simulink model "FixedWingModel"  (R2021a)
settings: configuration reference "ctrlConfigSet" (kept outside this file)
values from neighbouring files (symbols this model uses):
  ap = 0.01    [pathFollowingData.sldd]
  env = 0.0065    [pathFollowingData.sldd]
  sensors = 0.0    [pathFollowingData.sldd]
  uavParam = 2.795    [pathFollowingData.sldd]
undefined symbols (not defined in the file or in its folder): DiscIntNeverNeededParam, Earth, WGS84
libraries: simulink x24, mbdriLib x21, pid_lib x1, simulink_need_slupdate x1, aerolibconvert2 x1, aerolibtransform2 x1, uavalgslib x1
(part 1 of 2)
settings Model: DataDictionary=pathFollowingData.sldd  Creator=The MathWorks, Inc.  LastModifiedBy=saslab
settings ConfigSetRef: SourceName=ctrlConfigSet

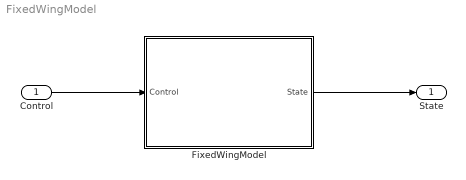
== system FixedWingModel ==
  Control : Inport  OutDataTypeStr=Bus: FixedWingControlBus  BusOutputAsStruct=on
  FixedWingModel : Subsystem  Variant=on
  State : Outport  OutDataTypeStr=Bus: FixedWingStateBus  VectorParamsAs1DForOutWhenUnconnected=off  BusOutputAsStruct=on
  wires:
  Control/1 -> FixedWingModel/1(Control)
  FixedWingModel/1(State) -> State/1

== system FixedWingModel/FixedWingModel ==
  Control : Inport
  HighFidelity : Subsystem  VariantControl=useHighFidelity == 1
  LowFidelity : Subsystem  VariantControl=useHighFidelity == 0
  State : Outport  VectorParamsAs1DForOutWhenUnconnected=off

== system FixedWingModel/FixedWingModel/HighFidelity ==
  Control : Inport
  Constant : Constant  Value=uavParam.ic.gsLL  OutDataTypeStr=single
  Constant1 : Constant  Value=uavParam.ic.Pos_0(3)  OutDataTypeStr=single
  ControlConversion : Subsystem
  FixedWingNoWindNoNoise : Subsystem
  Mux : Mux  Inputs=2
  StateConversion : Subsystem
  Terminator : Terminator
  State : Outport  VectorParamsAs1DForOutWhenUnconnected=off
  wires:
  Mux/1 -> FixedWingNoWindNoNoise/2(InitialPoint)
  Constant1/1 -> Mux/2
  Constant/1 -> Mux/1
  Control/1 -> ControlConversion/1(In1)
  FixedWingNoWindNoNoise/1(APStatus) -> Terminator/1
  FixedWingNoWindNoNoise/2(UAVStates) -> StateConversion/1(In1)
  StateConversion/1(Out1) -> State/1
  ControlConversion/1(Out1) -> FixedWingNoWindNoNoise/1(ControlCmd)

== system FixedWingModel/FixedWingModel/LowFidelity ==
  Control : Inport
  Bus Creator1 : BusCreator  Inputs=4  OutDataTypeStr=Bus: FixedWingEnvironmentBus  NonVirtualBus=on
  Constant : Constant  Value=0
  Constant1 : Constant  Value=0
  Constant2 : Constant  Value=0
  Constant5 : Constant  Value=env.ISA_g
  Fixed Wing UAV Guidance Model : uavalgslib/Guidance Model  ModelType=FixedWingGuidance  SpecifiedDataType=double  SimulateUsing=Code generation  InitialWorldPositionMultirotor=[0; 0; 0]  InitialWorldVelocityMultirotor=[0; 0; 0]  InitialEulerZYXMultirotor=[0; 0; 0]  InitialBodyAngularRateRPYMultirotor=[0; 0; 0]  InitialThrustMultirotor=0  InitialNorthFixedWing=1.882141015625000e+04  InitialEastFixedWing=-1.784960546875000e+04  InitialHeightFixedWing=2.037800048828125e+03  InitialAirSpeedFixedWing=30  InitialHeadingAngleFixedWing=1.9  InitialFlightPathAngleFixedWing=0  InitialRollAngleFixedWing=0  InitialRollAngleRateFixedWing=0  PDRollMultirotor=[3402.97,116.67]  PDPitchMultirotor=[3402.97, 116.67]  PYawRateMultirotor=1950  PThrustMultirotor=3900  MassMultirotor=0.1  PHeightFixedWing=0.78  PHeadingAngleFixedWing=3.9  PFlightPathAngleFixedWing=3.9  PDRollFixedWing="[5.4448      4.6668]"  PAirSpeedFixedWing=7.8  FlightPathAngleLimitsFixedWing=[-pi/4, pi/4]  StateBusName='FixedWingStateBus'  ControlBusName='FixedWingControlBus'  EnvironmentBusName='FixedWingEnvironmentBus'  DataType=double
      settings: SourceProductBaseCode=UV
  State : Outport  VectorParamsAs1DForOutWhenUnconnected=off
  wires:
  Constant5/1 -> Bus Creator1/4  "Gravity"
  Constant1/1 -> Bus Creator1/2  "WindEast"
  Bus Creator1/1 -> Fixed Wing UAV Guidance Model/2
  Control/1 -> Fixed Wing UAV Guidance Model/1
  Constant/1 -> Bus Creator1/1  "WindNorth"
  Fixed Wing UAV Guidance Model/1 -> State/1
  Constant2/1 -> Bus Creator1/3  "WindDown"

== system FixedWingModel/FixedWingModel/HighFidelity/ControlConversion ==
  In1 : Inport
  Bus Creator : BusCreator  Inputs=3  OutDataTypeStr=Bus: midLevelControlBus  NonVirtualBus=on
  Bus Selector : BusSelector  OutputSignals=Height,AirSpeed,RollAngle
  Data Type Conversion : DataTypeConversion
  Data Type Conversion1 : DataTypeConversion
  Data Type Conversion2 : DataTypeConversion
  Out1 : Outport  VectorParamsAs1DForOutWhenUnconnected=off
  wires:
  In1/1 -> Bus Selector/1
  Bus Creator/1 -> Out1/1
  Bus Selector/1 -> Data Type Conversion/1  "<Height>"
  Bus Selector/2 -> Data Type Conversion1/1  "<AirSpeed>"
  Data Type Conversion/1 -> Bus Creator/1  "h_c"
  Data Type Conversion1/1 -> Bus Creator/2  "U_c"
  Bus Selector/3 -> Data Type Conversion2/1  "<RollAngle>"
  Data Type Conversion2/1 -> Bus Creator/3  "phi_c"

== system FixedWingModel/FixedWingModel/HighFidelity/FixedWingNoWindNoNoise ==
  ControlCmd : Inport  OutDataTypeStr=Bus: midLevelControlBus
  InitialPoint : Inport  Port=2  PortDimensions=3
  AP Config Parameters : Subsystem
  Constant : Constant  Value=0  OutDataTypeStr=Inherit: Inherit via back propagation
  Constant1 : Constant  Value=0  OutDataTypeStr=Inherit: Inherit via back propagation
  Constant2 : Constant  Value=0  OutDataTypeStr=Inherit: Inherit via back propagation
  FixedWingAutopilotModel : Subsystem
  APStatus : Outport  VectorParamsAs1DForOutWhenUnconnected=off
  UAVStates : Outport  Port=2  VectorParamsAs1DForOutWhenUnconnected=off
  wires:
  AP Config Parameters/1(apConfigParams) -> FixedWingAutopilotModel/5(ControlGains)
  Constant2/1 -> FixedWingAutopilotModel/6(ManualMode)
  Constant/1 -> FixedWingAutopilotModel/3(WindSwitch)
  FixedWingAutopilotModel/1(apStatus) -> APStatus/1
  Constant1/1 -> FixedWingAutopilotModel/4(NoiseSwitch)
  InitialPoint/1 -> FixedWingAutopilotModel/1(InitialLongtitudeLatitude)
  ControlCmd/1 -> FixedWingAutopilotModel/2(MidLevelCmd)
  FixedWingAutopilotModel/2(UAVState) -> UAVStates/1

== system FixedWingModel/FixedWingModel/HighFidelity/StateConversion ==
  In1 : Inport
  Bus Creator : BusCreator  Inputs=8  OutDataTypeStr=Bus: FixedWingStateBus  NonVirtualBus=on
  Bus Selector : BusSelector  OutputSignals=X_e,airspeed,V_e,Euler,pqr
  Demux : Demux  Outputs=3
  Gain : Gain  Gain=-1
  Gain1 : Gain
  Selector : Selector  InputPortWidth=3  IndexOptions=Index vector (dialog)  Indices=[1]  OutputSizes=1
  Selector1 : Selector  InputPortWidth=3  IndexOptions=Index vector (dialog)  Indices=[1]  OutputSizes=1
  Subsystem : Subsystem
  Out1 : Outport  VectorParamsAs1DForOutWhenUnconnected=off
  wires:
  Bus Creator/1 -> Out1/1
  Gain1/1 -> Bus Creator/4  "AirSpeed"
  Subsystem/2(FlightPath) -> Bus Creator/6  "FlightPathAngle"
  Bus Selector/2 -> Gain1/1  "<airspeed>"
  Selector/1 -> Bus Creator/7  "RollAngle"
  Bus Selector/4 -> Selector/1  "<Euler>"
  Bus Selector/1 -> Demux/1  "<X_e>"
  Bus Selector/3 -> Subsystem/1(Ve)  "<V_e>"
  Demux/2 -> Bus Creator/2  "East"
  Bus Selector/5 -> Selector1/1  "<pqr>"
  Subsystem/1(Heading) -> Bus Creator/5  "HeadingAngle"
  Demux/1 -> Bus Creator/1  "North"
  Demux/3 -> Gain/1
  Selector1/1 -> Bus Creator/8  "RollAngleRate"
  Gain/1 -> Bus Creator/3  "Height"
  In1/1 -> Bus Selector/1

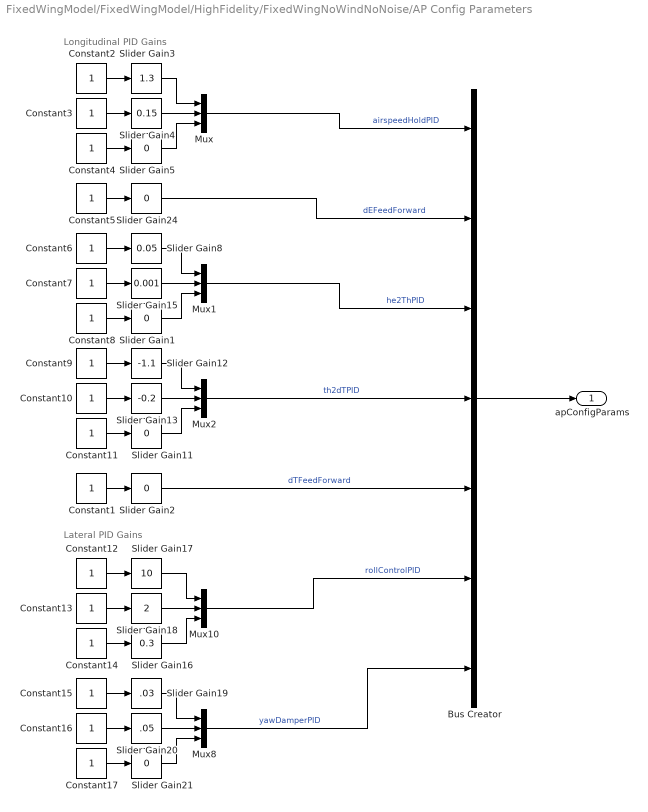
== system FixedWingModel/FixedWingModel/HighFidelity/FixedWingNoWindNoNoise/AP Config Parameters ==
  note: Longitudinal PID Gains
  note: Lateral PID Gains
  Bus Creator : BusCreator  Inputs=7  OutDataTypeStr=Bus: apConfigParamsBus
  Constant{1..17} (17 alike) : Constant  OutDataTypeStr=single  SampleTime=ap.apSampleTime
      settings: AttributesFormatString=%<Value>
  Mux{,1..2,8,10} (5 alike) : Mux  Inputs=3
  Slider Gain1 : simulink/Math Operations/Slider Gain  gain=0  low=-20  high=20
  Slider Gain11 : simulink/Math Operations/Slider Gain  gain=0  low=-0.1  high=0
  Slider Gain12 : simulink/Math Operations/Slider Gain  gain=-1.1  low=-2  high=0.5
  Slider Gain13 : simulink/Math Operations/Slider Gain  gain=-0.2  low=-0.2  high=0
  Slider Gain15 : simulink/Math Operations/Slider Gain  gain=0.001  low=-20  high=20
  Slider Gain16 : simulink/Math Operations/Slider Gain  gain=0.3  low=-0.1  high=5
  Slider Gain17 : simulink/Math Operations/Slider Gain  gain=10  low=-0.1  high=50
  Slider Gain18 : simulink/Math Operations/Slider Gain  gain=2  low=0  high=2
  Slider Gain19 : simulink/Math Operations/Slider Gain  gain=.03  low=-20  high=20
  Slider Gain2 : simulink/Math Operations/Slider Gain  gain=0  low=-0.1  high=5
  Slider Gain20 : simulink/Math Operations/Slider Gain  gain=.05  low=-20  high=20
  Slider Gain21 : simulink/Math Operations/Slider Gain  gain=0  low=-20  high=20
  Slider Gain24 : simulink/Math Operations/Slider Gain  gain=0  low=-0.1  high=5
  Slider Gain3 : simulink/Math Operations/Slider Gain  gain=1.3  low=-0.5  high=4.5
  Slider Gain4 : simulink/Math Operations/Slider Gain  gain=0.15  low=-20  high=20
  Slider Gain5 : simulink/Math Operations/Slider Gain  gain=0  low=-20  high=20
  Slider Gain8 : simulink/Math Operations/Slider Gain  gain=0.05  low=-20  high=20
  apConfigParams : Outport  OutDataTypeStr=Bus: apConfigParamsBus  VectorParamsAs1DForOutWhenUnconnected=off
  wires:
  Mux8/1 -> Bus Creator/7  "yawDamperPID"
  Slider Gain21/1 -> Mux8/3
  Slider Gain19/1 -> Mux8/1
  Slider Gain20/1 -> Mux8/2
  Constant17/1 -> Slider Gain21/1
  Constant16/1 -> Slider Gain20/1
  Constant15/1 -> Slider Gain19/1
  Mux10/1 -> Bus Creator/6  "rollControlPID"
  Slider Gain16/1 -> Mux10/3
  Slider Gain17/1 -> Mux10/1
  Slider Gain18/1 -> Mux10/2
  Constant14/1 -> Slider Gain16/1
  Constant13/1 -> Slider Gain18/1
  Constant12/1 -> Slider Gain17/1
  Constant1/1 -> Slider Gain2/1
  Slider Gain1/1 -> Mux1/3
  Slider Gain15/1 -> Mux1/2
  Mux2/1 -> Bus Creator/4  "th2dTPID"
  Slider Gain11/1 -> Mux2/3
  Slider Gain12/1 -> Mux2/1
  Slider Gain13/1 -> Mux2/2
  Constant11/1 -> Slider Gain11/1
  Constant10/1 -> Slider Gain13/1
  Constant9/1 -> Slider Gain12/1
  Mux1/1 -> Bus Creator/3  "he2ThPID"
  Slider Gain8/1 -> Mux1/1
  Constant8/1 -> Slider Gain1/1
  Constant7/1 -> Slider Gain15/1
  Constant6/1 -> Slider Gain8/1
  Slider Gain24/1 -> Bus Creator/2  "dEFeedForward"
  Constant5/1 -> Slider Gain24/1
  Mux/1 -> Bus Creator/1  "airspeedHoldPID"
  Slider Gain5/1 -> Mux/3
  Slider Gain3/1 -> Mux/1
  Slider Gain4/1 -> Mux/2
  Constant4/1 -> Slider Gain5/1
  Constant3/1 -> Slider Gain4/1
  Constant2/1 -> Slider Gain3/1
  Bus Creator/1 -> apConfigParams/1
  Slider Gain2/1 -> Bus Creator/5  "dTFeedForward"

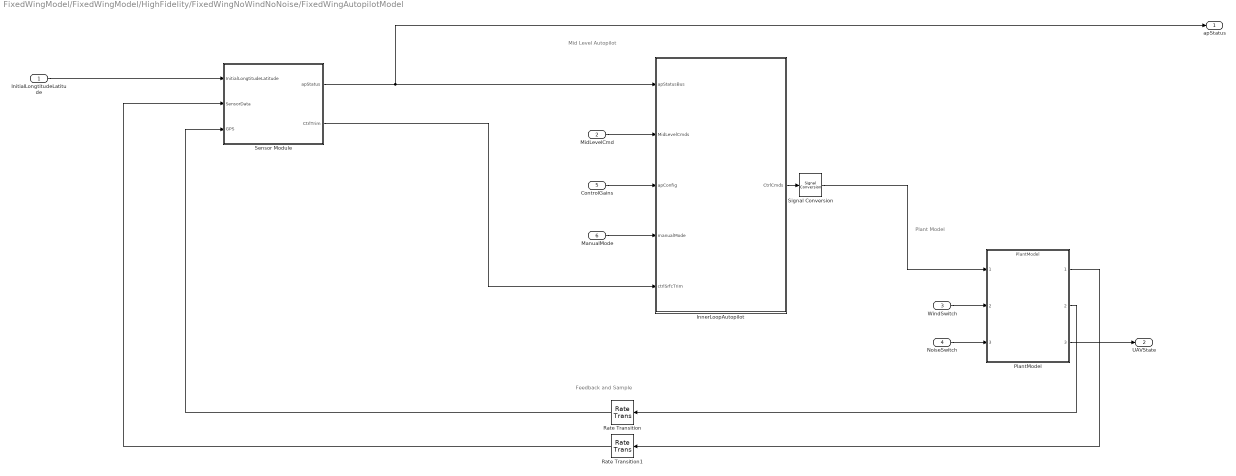
== system FixedWingModel/FixedWingModel/HighFidelity/FixedWingNoWindNoNoise/FixedWingAutopilotModel ==
  note: Mid Level Autopilot
  note: Plant Model
  note: Feedback and Sample
  InitialLongtitudeLatitude : Inport  SampleTime=[0.01,0]  BusOutputAsStruct=on
  MidLevelCmd : Inport  Port=2  OutDataTypeStr=Bus: midLevelControlBus
  WindSwitch : Inport  Port=3
  NoiseSwitch : Inport  Port=4
  ControlGains : Inport  Port=5
  ManualMode : Inport  Port=6
  InnerLoopAutopilot : Subsystem  TreatAsAtomicUnit=on
  PlantModel : ModelReference  ModelNameDialog=PlantModel  SimulationMode=Normal  ModelReferenceVersion=2.0
  Rate Transition : RateTransition  OutPortSampleTime=ap.apSampleTime
  Rate Transition1 : RateTransition  OutPortSampleTime=ap.apSampleTime
      settings: AttributesFormatString=%<OutPortSampleTime>
  Sensor Module : Subsystem
  Signal Conversion : SignalConversion  ConversionOutput=Nonvirtual bus  OutDataTypeStr=Bus: ctrlCmdsBus  OverrideOpt=off
  apStatus : Outport  VectorParamsAs1DForOutWhenUnconnected=off
  UAVState : Outport  Port=2  VectorParamsAs1DForOutWhenUnconnected=off
  wires:
  InitialLongtitudeLatitude/1 -> Sensor Module/1(InitialLongtitudeLatitude)
  MidLevelCmd/1 -> InnerLoopAutopilot/2(MidLevelCmds)
  PlantModel/1 -> Rate Transition1/1
  InnerLoopAutopilot/1(CtrlCmds) -> Signal Conversion/1
  Signal Conversion/1 -> PlantModel/1
  NoiseSwitch/1 -> PlantModel/3
  ManualMode/1 -> InnerLoopAutopilot/4(manualMode)
  ControlGains/1 -> InnerLoopAutopilot/3(apConfig)
  WindSwitch/1 -> PlantModel/2
  PlantModel/3 -> UAVState/1
  PlantModel/2 -> Rate Transition/1
  Rate Transition/1 -> Sensor Module/3(GPS)
  Rate Transition1/1 -> Sensor Module/2(SensorData)
  Sensor Module/1(apStatus) -> apStatus/1, InnerLoopAutopilot/1(apStatusBus)
  Sensor Module/2(CtrlTrim) -> InnerLoopAutopilot/5(ctrlSrfcTrim)

== system FixedWingModel/FixedWingModel/HighFidelity/StateConversion/Subsystem ==
  Ve : Inport
  Add : Sum
  Atan : Trigonometry  Operator=atan2
  Atan1 : Trigonometry  Operator=atan2
  Demux : Demux  Outputs=2
  Selector : Selector  InputPortWidth=3  IndexOptions=Index vector (dialog)  Indices=[2 1]  OutputSizes=1
  Selector1 : Selector  InputPortWidth=3  IndexOptions=Index vector (dialog)  Indices=[3]  OutputSizes=1
  Sqrt : Sqrt  SaturateOnIntegerOverflow=on
  Square : Math  Operator=square  SignedPower=on  SaturateOnIntegerOverflow=on
  Square1 : Math  Operator=square  SignedPower=on  SaturateOnIntegerOverflow=on
  Heading : Outport  VectorParamsAs1DForOutWhenUnconnected=off
  FlightPath : Outport  Port=2  VectorParamsAs1DForOutWhenUnconnected=off
  wires:
  Demux/1 -> Square/1, Atan/1
  Demux/2 -> Square1/1, Atan/2
  Selector/1 -> Demux/1
  Ve/1 -> Selector1/1, Selector/1
  Atan/1 -> Heading/1
  Atan1/1 -> FlightPath/1
  Selector1/1 -> Atan1/1
  Add/1 -> Sqrt/1
  Sqrt/1 -> Atan1/2
  Square/1 -> Add/1
  Square1/1 -> Add/2

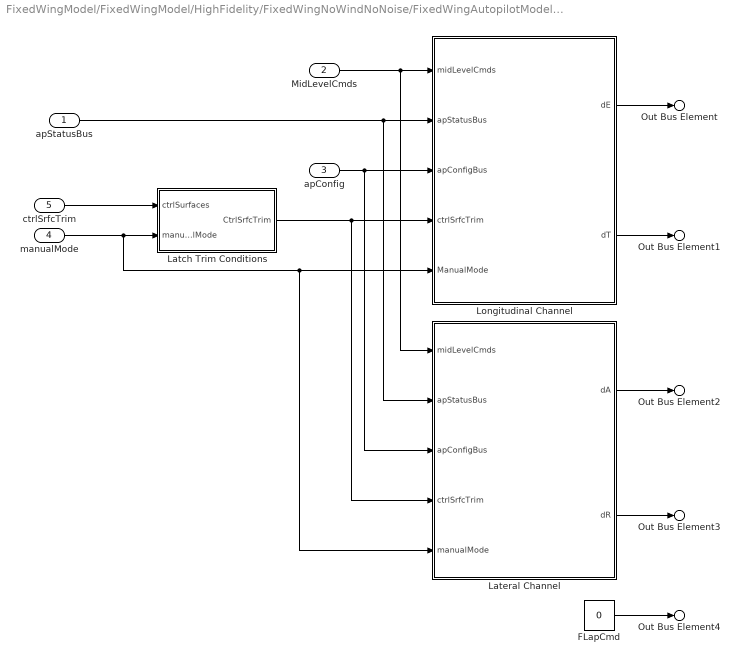
== system FixedWingModel/FixedWingModel/HighFidelity/FixedWingNoWindNoNoise/FixedWingAutopilotModel/InnerLoopAutopilot ==
  apStatusBus : Inport  OutDataTypeStr=Bus: apStatusBus
  MidLevelCmds : Inport  Port=2
  apConfig : Inport  Port=3  OutDataTypeStr=Bus: apConfigParamsBus
  manualMode : Inport  Port=4
  ctrlSrfcTrim : Inport  Port=5
  FLapCmd : Constant  Value=0  OutDataTypeStr=single  SampleTime=ap.apSampleTime
      settings: AttributesFormatString=%<Value>
  Latch Trim Conditions : Subsystem
  Lateral Channel : Subsystem  TreatAsAtomicUnit=on
  Longitudinal Channel : Subsystem  TreatAsAtomicUnit=on
  Out Bus Element : Outport  VectorParamsAs1DForOutWhenUnconnected=off  PortName=CtrlCmds  Element=elevatorCmd
  Out Bus Element1 : Outport  VectorParamsAs1DForOutWhenUnconnected=off  PortName=CtrlCmds  Element=throttleCmd
  Out Bus Element2 : Outport  VectorParamsAs1DForOutWhenUnconnected=off  PortName=CtrlCmds  Element=aileronCmd
  Out Bus Element3 : Outport  VectorParamsAs1DForOutWhenUnconnected=off  PortName=CtrlCmds  Element=rudderCmd
  Out Bus Element4 : Outport  VectorParamsAs1DForOutWhenUnconnected=off  PortName=CtrlCmds  Element=flapCmd
  wires:
  manualMode/1 -> Latch Trim Conditions/2(manualMode), Lateral Channel/5(manualMode), Longitudinal Channel/5(ManualMode)
  Latch Trim Conditions/1(CtrlSrfcTrim) -> Lateral Channel/4(ctrlSrfcTrim), Longitudinal Channel/4(ctrlSrfcTrim)
  ctrlSrfcTrim/1 -> Latch Trim Conditions/1(ctrlSurfaces)
  apConfig/1 -> Lateral Channel/3(apConfigBus), Longitudinal Channel/3(apConfigBus)
  FLapCmd/1 -> Out Bus Element4/1
  Lateral Channel/2(dR) -> Out Bus Element3/1
  Lateral Channel/1(dA) -> Out Bus Element2/1
  Longitudinal Channel/2(dT) -> Out Bus Element1/1
  Longitudinal Channel/1(dE) -> Out Bus Element/1
  apStatusBus/1 -> Lateral Channel/2(apStatusBus), Longitudinal Channel/2(apStatusBus)
  MidLevelCmds/1 -> Lateral Channel/1(midLevelCmds), Longitudinal Channel/1(midLevelCmds)

== system FixedWingModel/FixedWingModel/HighFidelity/FixedWingNoWindNoNoise/FixedWingAutopilotModel/Sensor Module ==
  InitialLongtitudeLatitude : Inport
  SensorData : Inport  Port=2
  GPS : Inport  Port=3
  Position Filter : Subsystem  TreatAsAtomicUnit=on
  SensorConditioning : Subsystem  TreatAsAtomicUnit=on
  apStatusCreation : Subsystem
  apStatus : Outport  VectorParamsAs1DForOutWhenUnconnected=off
  CtrlTrim : Outport  Port=2  VectorParamsAs1DForOutWhenUnconnected=off
  wires:
  InitialLongtitudeLatitude/1 -> Position Filter/3(InitialLongtitudeLatitude)
  SensorConditioning/1(FilteredSensorData) -> apStatusCreation/3(FilteredSensorData), Position Filter/1(FilteredSensorData)
  SensorConditioning/2(CtrlSurfaces) -> CtrlTrim/1
  GPS/1 -> apStatusCreation/2(GPSData), Position Filter/2(GPSData)
  SensorData/1 -> SensorConditioning/1(RawSensorData)
  apStatusCreation/1(apStatus) -> apStatus/1
  Position Filter/1(PosVel_hat) -> apStatusCreation/1(PosVel_hat)

== system FixedWingModel/FixedWingModel/HighFidelity/FixedWingNoWindNoNoise/FixedWingAutopilotModel/InnerLoopAutopilot/Latch Trim Conditions ==
  ctrlSurfaces : Inport
  manualMode : Inport  Port=2
  Compare To Constant : simulink/Logic and Bit Operations/Compare To Constant  relop===  const=1  OutDataTypeStr=boolean
  Latch Control Surfaces Trim from any mode : Subsystem  TreatAsAtomicUnit=on
  CtrlSrfcTrim : Outport  VectorParamsAs1DForOutWhenUnconnected=off
  wires:
  manualMode/1 -> Compare To Constant/1
  Latch Control Surfaces Trim from any mode/1(Trim) -> CtrlSrfcTrim/1
  Compare To Constant/1 -> Latch Control Surfaces Trim from any mode/Trigger
  ctrlSurfaces/1 -> Latch Control Surfaces Trim from any mode/1(ctrlSurfaces)

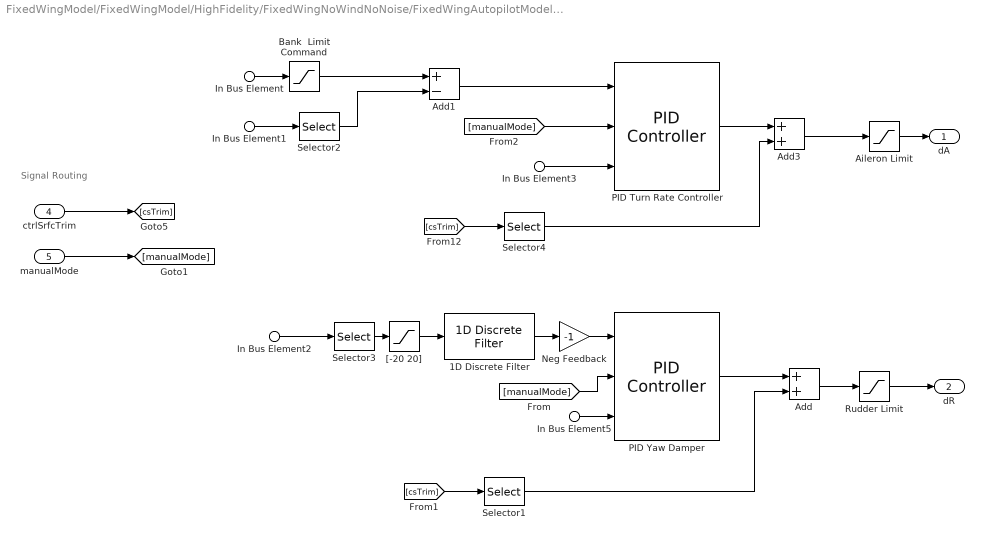
== system FixedWingModel/FixedWingModel/HighFidelity/FixedWingNoWindNoNoise/FixedWingAutopilotModel/InnerLoopAutopilot/Lateral Channel ==
  note: Signal Routing
  In Bus Element : Inport  PortName=midLevelCmds  Element=phi_c
  In Bus Element1 : Inport  Port=2  PortName=apStatusBus  Element=Euler
  In Bus Element2 : Inport  Port=2  PortName=apStatusBus  Element=Ab
  In Bus Element3 : Inport  Port=3  PortName=apConfigBus  Element=rollControlPID
  In Bus Element5 : Inport  Port=3  PortName=apConfigBus  Element=yawDamperPID
  ctrlSrfcTrim : Inport  Port=4
  manualMode : Inport  Port=5
  1D Discrete Filter : mbdriLib/Filtering/1D Discrete Filter  bw=10  TSample=ap.apSampleTime
      settings: AttributesFormatString=Fc = 10
  Add : Sum  OutDataTypeStr=single
  Add1 : Sum  Inputs=+-  OutDataTypeStr=single
  Add3 : Sum  OutDataTypeStr=single
  Aileron Limit : Saturate  UpperLimit=ap.control.daLimit  LowerLimit=-ap.control.daLimit
      settings: AttributesFormatString="[%<LowerLimit>  %<UpperLimit>]"
  Bank  Limit Command : Saturate  UpperLimit=ap.control.phi_cLimit  LowerLimit=-ap.control.phi_cLimit
      settings: AttributesFormatString="[%<LowerLimit>  %<UpperLimit>]"
  Neg Feedback : Gain  Gain=-1  OutDataTypeStr=float('double')
      settings: AttributesFormatString=%<Gain>
  PID Turn Rate Controller : mbdriLib/Control/PID Controller  Tsample=ap.apSampleTime  Ndelay=ap.control.derivativesConstant  upperSaturationLimit=ap.control.daLimit  lowerSaturationLimit=-ap.control.daLimit
  PID Yaw Damper : mbdriLib/Control/PID Controller  Tsample=ap.apSampleTime  Ndelay=ap.control.derivativesConstant  upperSaturationLimit=ap.control.drLimit  lowerSaturationLimit=-ap.control.drLimit
  Rudder Limit : Saturate  UpperLimit=ap.control.drLimit  LowerLimit=-ap.control.drLimit
      settings: AttributesFormatString="[%<LowerLimit>  %<UpperLimit>]"
  Selector1 : Selector  InputPortWidth=5  IndexOptions=Index vector (dialog)  Indices=[3]  OutputSizes=1
  Selector2 : Selector  InputPortWidth=3  IndexOptions=Index vector (dialog)  Indices=[1]  OutputSizes=1
  Selector3 : Selector  InputPortWidth=3  IndexOptions=Index vector (dialog)  Indices=[2]  OutputSizes=1
  Selector4 : Selector  InputPortWidth=5  IndexOptions=Index vector (dialog)  Indices=[2]  OutputSizes=1
  "[-20 20]" : Saturate  UpperLimit=20  LowerLimit=-20
      settings: AttributesFormatString="[%<LowerLimit>  %<UpperLimit>]"
  dA : Outport  VectorParamsAs1DForOutWhenUnconnected=off
  dR : Outport  Port=2  VectorParamsAs1DForOutWhenUnconnected=off
  wires:
  [manualMode] -> PID Turn Rate Controller/2
  In Bus Element2/1 -> Selector3/1
  Selector3/1 -> "[-20 20]"/1
  [manualMode] -> PID Yaw Damper/2
  In Bus Element5/1 -> PID Yaw Damper/3
  [csTrim] -> Selector1/1
  [csTrim] -> Selector4/1
  Selector2/1 -> Add1/2
  In Bus Element1/1 -> Selector2/1
  Bank  Limit Command/1 -> Add1/1
  ctrlSrfcTrim/1 -> [csTrim]
  Selector1/1 -> Add/2
  1D Discrete Filter/1 -> Neg Feedback/1
  "[-20 20]"/1 -> 1D Discrete Filter/1
  Selector4/1 -> Add3/2
  Neg Feedback/1 -> PID Yaw Damper/1
  In Bus Element/1 -> Bank  Limit Command/1
  Add1/1 -> PID Turn Rate Controller/1
  Aileron Limit/1 -> dA/1
  PID Turn Rate Controller/1 -> Add3/1
  Add3/1 -> Aileron Limit/1
  In Bus Element3/1 -> PID Turn Rate Controller/3
  PID Yaw Damper/1 -> Add/1
  Add/1 -> Rudder Limit/1
  Rudder Limit/1 -> dR/1
  manualMode/1 -> [manualMode]

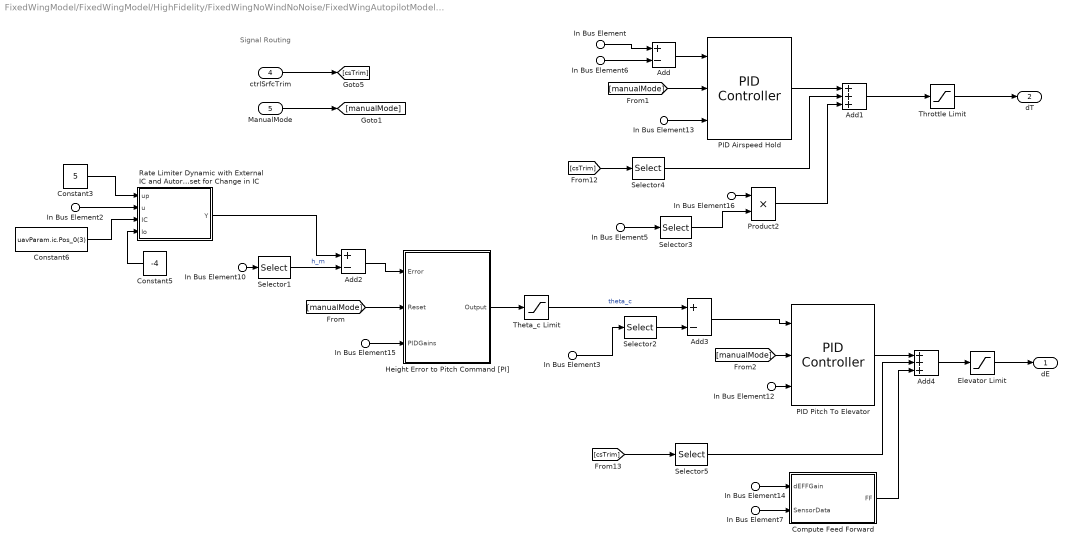
== system FixedWingModel/FixedWingModel/HighFidelity/FixedWingNoWindNoNoise/FixedWingAutopilotModel/InnerLoopAutopilot/Longitudinal Channel ==
  note: Signal Routing
  In Bus Element : Inport  PortName=midLevelCmds  Element=U_c
  In Bus Element2 : Inport  PortName=midLevelCmds  Element=h_c
  In Bus Element7 : Inport  Port=2  PortName=apStatusBus
  In Bus Element6 : Inport  Port=2  PortName=apStatusBus  Element=ias
  In Bus Element10 : Inport  Port=2  PortName=apStatusBus  Element=Xe
  In Bus Element3 : Inport  Port=2  PortName=apStatusBus  Element=Euler
  In Bus Element5 : Inport  Port=2  PortName=apStatusBus  Element=Euler
  In Bus Element12 : Inport  Port=3  PortName=apConfigBus  Element=th2dTPID
  In Bus Element13 : Inport  Port=3  PortName=apConfigBus  Element=airspeedHoldPID
  In Bus Element16 : Inport  Port=3  PortName=apConfigBus  Element=dEFeedForward
  In Bus Element15 : Inport  Port=3  PortName=apConfigBus  Element=he2ThPID
  In Bus Element14 : Inport  Port=3  PortName=apConfigBus  Element=dTFeedForward
  ctrlSrfcTrim : Inport  Port=4
  ManualMode : Inport  Port=5
  Add : Sum  Inputs=+-
  Add1 : Sum  Inputs=3  OutDataTypeStr=single
  Add2 : Sum  Inputs=+-  OutDataTypeStr=single
  Add3 : Sum  Inputs=+-  OutDataTypeStr=single
  Add4 : Sum  Inputs=3  OutDataTypeStr=single
  Compute Feed Forward : Subsystem
  Constant3 : Constant  Value=5  OutDataTypeStr=single
      settings: AttributesFormatString=%<Value>
  Constant5 : Constant  Value=-4  OutDataTypeStr=single
      settings: AttributesFormatString=%<Value>
  Constant6 : Constant  Value=uavParam.ic.Pos_0(3)  OutDataTypeStr=single
      settings: AttributesFormatString=%<Value>
  Elevator Limit : Saturate  UpperLimit=ap.control.deLimit  LowerLimit=-ap.control.deLimit
      settings: AttributesFormatString="[%<LowerLimit>  %<UpperLimit>]"
  Height Error to Pitch Command [PI] : Subsystem  mask(PID){Tsample=ap.apSampleTime, Ndelay=ap.control.derivativesConstant, upperSaturationLimit=ap.control.the_cLimit, lowerSaturationLimit=-ap.control.the_cLimit}
      mask prompts: Tsample "Sample Time"; Ndelay "Integer delays for de/dt"; upperSaturationLimit "Upper Saturation Limit"; lowerSaturationLimit "Lower Saturation Limit"
      mask help: PID controller block with anti-windup and saturation limits. Implemented as a discrete forwardl integration which stops integrating when the output is saturated. Derivative is implemented as a numerical derivative with N integer delays to smooth output.
      mask Display:
      | disp('PI')
      | port_label('input',1,'error')
      | port_label('input',3,'gains')
      | port_label('input',2,'reset')
      | port_label('output',1,'output')
  PID Airspeed Hold : mbdriLib/Control/PID Controller  Tsample=ap.apSampleTime  Ndelay=ap.control.derivativesConstant  upperSaturationLimit=ap.control.dtLimit  lowerSaturationLimit=0
  PID Pitch To Elevator : mbdriLib/Control/PID Controller  Tsample=ap.apSampleTime  Ndelay=ap.control.derivativesConstant  upperSaturationLimit=ap.control.deLimit  lowerSaturationLimit=-ap.control.deLimit
  Product2 : Product  RndMeth=Zero
  Rate Limiter Dynamic with External IC and Autoreset for Change in IC : Subsystem
      mask Display:
      | plot([0.15 0.95],[.5 .5],[.5 .5],[0.05 0.95],0.05+0.9*[.2 .8],0.05+0.9*[0 1]);
      | port_label('output',1,'Y');
      | port_label('input',1,'up');
      | port_label('input',2,'u');
      | port_label('input',3,'IC');
      | port_label('input',4,'Lo');
  Selector1 : Selector  InputPortWidth=3  IndexOptions=Index vector (dialog)  Indices=[3]  OutputSizes=1
  Selector2 : Selector  InputPortWidth=3  IndexOptions=Index vector (dialog)  Indices=[2]  OutputSizes=1
  Selector3 : Selector  InputPortWidth=3  IndexOptions=Index vector (dialog)  Indices=[2]  OutputSizes=1
  Selector4 : Selector  InputPortWidth=5  IndexOptions=Index vector (dialog)  Indices=[1]  OutputSizes=1
  Selector5 : Selector  InputPortWidth=5  IndexOptions=Index vector (dialog)  Indices=[5]  OutputSizes=1
  Theta_c Limit : Saturate  UpperLimit=ap.control.the_cLimit  LowerLimit=-ap.control.the_cLimit  SampleTime=ap.apSampleTime
      settings: AttributesFormatString="[%<LowerLimit>  %<UpperLimit>]"
  Throttle Limit : Saturate  UpperLimit=ap.control.dtLimit  LowerLimit=0
      settings: AttributesFormatString="[%<LowerLimit>  %<UpperLimit>]"
  dE : Outport  VectorParamsAs1DForOutWhenUnconnected=off
  dT : Outport  Port=2  VectorParamsAs1DForOutWhenUnconnected=off
  wires:
  Selector5/1 -> Add4/2
  [csTrim] -> Selector5/1
  [manualMode] -> PID Pitch To Elevator/2
  [manualMode] -> PID Airspeed Hold/2
  Add4/1 -> Elevator Limit/1
  Elevator Limit/1 -> dE/1
  Throttle Limit/1 -> dT/1
  Selector4/1 -> Add1/2
  [csTrim] -> Selector4/1
  ctrlSrfcTrim/1 -> [csTrim]
  In Bus Element5/1 -> Selector3/1
  In Bus Element14/1 -> Compute Feed Forward/1(dEFFGain)
  In Bus Element16/1 -> Product2/1
  Product2/1 -> Add1/3
  Selector3/1 -> Product2/2
  In Bus Element12/1 -> PID Pitch To Elevator/3
  In Bus Element3/1 -> Selector2/1
  Selector2/1 -> Add3/2
  In Bus Element7/1 -> Compute Feed Forward/2(SensorData)
  In Bus Element10/1 -> Selector1/1
  In Bus Element/1 -> Add/1
  Add1/1 -> Throttle Limit/1
  Constant6/1 -> Rate Limiter Dynamic with External IC and Autoreset for Change in IC/3(IC)
  Constant5/1 -> Rate Limiter Dynamic with External IC and Autoreset for Change in IC/4(lo)
  Constant3/1 -> Rate Limiter Dynamic with External IC and Autoreset for Change in IC/1(up)
  In Bus Element15/1 -> Height Error to Pitch Command [PI]/3(PIDGains)
  In Bus Element13/1 -> PID Airspeed Hold/3
  In Bus Element6/1 -> Add/2
  Compute Feed Forward/1(FF) -> Add4/3
  Height Error to Pitch Command [PI]/1(Output) -> Theta_c Limit/1
  Theta_c Limit/1 -> Add3/1  "theta_c"
  Add3/1 -> PID Pitch To Elevator/1
  PID Pitch To Elevator/1 -> Add4/1
  [manualMode] -> Height Error to Pitch Command [PI]/2(Reset)
  Selector1/1 -> Add2/2  "h_m"
  Add2/1 -> Height Error to Pitch Command [PI]/1(Error)
  PID Airspeed Hold/1 -> Add1/1
  Add/1 -> PID Airspeed Hold/1
  In Bus Element2/1 -> Rate Limiter Dynamic with External IC and Autoreset for Change in IC/2(u)
  Rate Limiter Dynamic with External IC and Autoreset for Change in IC/1(Y) -> Add2/1
  ManualMode/1 -> [manualMode]

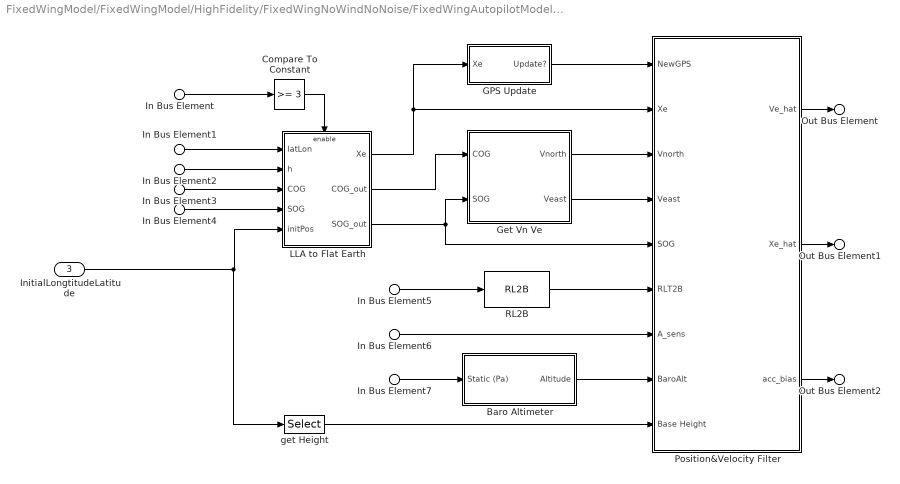
== system FixedWingModel/FixedWingModel/HighFidelity/FixedWingNoWindNoNoise/FixedWingAutopilotModel/Sensor Module/Position Filter ==
  In Bus Element5 : Inport  PortName=FilteredSensorData  Element=Euler
  In Bus Element6 : Inport  PortName=FilteredSensorData  Element=Ab
  In Bus Element7 : Inport  PortName=FilteredSensorData  Element=baro
  In Bus Element : Inport  Port=2  PortName=GPSData  Element=gps_fix
  In Bus Element1 : Inport  Port=2  PortName=GPSData  Element=gps_latLon
  In Bus Element2 : Inport  Port=2  PortName=GPSData  Element=gps_h
  In Bus Element3 : Inport  Port=2  PortName=GPSData  Element=gps_cog
  In Bus Element4 : Inport  Port=2  PortName=GPSData  Element=gps_sog
  InitialLongtitudeLatitude : Inport  Port=3
  Baro Altimeter : Subsystem
  Compare To Constant : simulink/Logic and Bit Operations/Compare To Constant  relop=>=  const=3  OutDataTypeStr=boolean
  GPS Update : Subsystem  mask{T=ap.apSampleTime}
      mask prompts: T "Sample Time"
  Get Vn Ve : Subsystem
  LLA to Flat Earth : Subsystem
  Position&Velocity Filter : Subsystem
  RL2B : mbdriLib/Coordinates/RL2B  SystemSampleTime=-1  VariantActivationTime=update diagram  Latency=0  AutoFrameSizeCalculation=off
  get Height : Selector  InputPortWidth=3  IndexOptions=Index vector (dialog)  Indices=[3]  OutputSizes=1
  Out Bus Element : Outport  VectorParamsAs1DForOutWhenUnconnected=off  PortName=PosVel_hat  Element=Ve_hat
  Out Bus Element1 : Outport  VectorParamsAs1DForOutWhenUnconnected=off  PortName=PosVel_hat  Element=Xe_hat
  Out Bus Element2 : Outport  VectorParamsAs1DForOutWhenUnconnected=off  PortName=PosVel_hat  Element=Ab_bias_hat
  wires:
  LLA to Flat Earth/1(Xe) -> Position&Velocity Filter/2(Xe), GPS Update/1(Xe)
  get Height/1 -> Position&Velocity Filter/9(Base Height)
  In Bus Element6/1 -> Position&Velocity Filter/7(A_sens)
  RL2B/1 -> Position&Velocity Filter/6(RLT2B)
  In Bus Element5/1 -> RL2B/1
  In Bus Element7/1 -> Baro Altimeter/1(Static (Pa))
  Baro Altimeter/1(Altitude) -> Position&Velocity Filter/8(BaroAlt)
  Get Vn Ve/2(Veast) -> Position&Velocity Filter/4(Veast)
  Get Vn Ve/1(Vnorth) -> Position&Velocity Filter/3(Vnorth)
  GPS Update/1(Update?) -> Position&Velocity Filter/1(NewGPS)
  InitialLongtitudeLatitude/1 -> LLA to Flat Earth/5(initPos), get Height/1
  In Bus Element4/1 -> LLA to Flat Earth/4(SOG)
  In Bus Element3/1 -> LLA to Flat Earth/3(COG)
  In Bus Element2/1 -> LLA to Flat Earth/2(h)
  In Bus Element1/1 -> LLA to Flat Earth/1(latLon)
  Compare To Constant/1 -> LLA to Flat Earth/Enable
  In Bus Element/1 -> Compare To Constant/1
  Position&Velocity Filter/2(Xe_hat) -> Out Bus Element1/1
  Position&Velocity Filter/1(Ve_hat) -> Out Bus Element/1
  Position&Velocity Filter/3(acc_bias) -> Out Bus Element2/1
  LLA to Flat Earth/2(COG_out) -> Get Vn Ve/1(COG)
  LLA to Flat Earth/3(SOG_out) -> Get Vn Ve/2(SOG), Position&Velocity Filter/5(SOG)

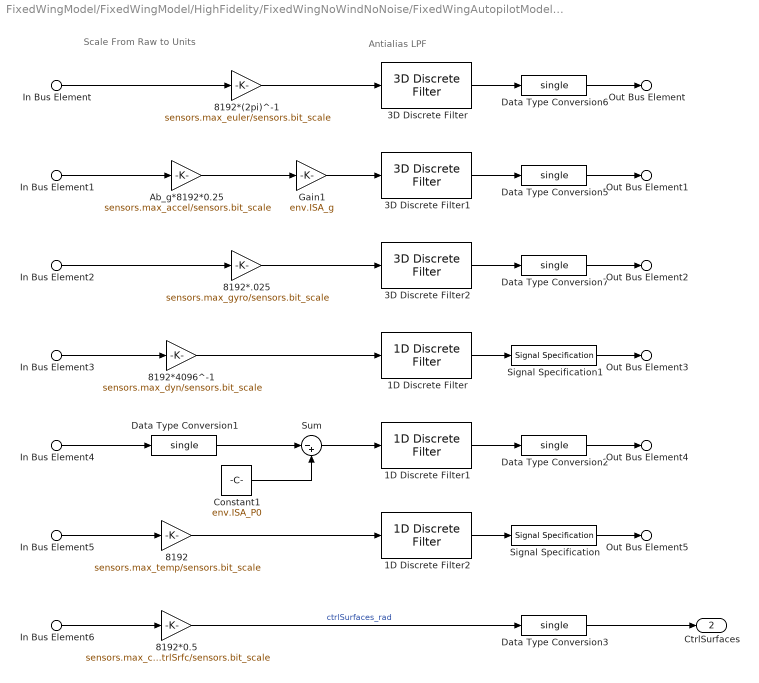
== system FixedWingModel/FixedWingModel/HighFidelity/FixedWingNoWindNoNoise/FixedWingAutopilotModel/Sensor Module/SensorConditioning ==
  note: Antialias LPF
  note: Scale From Raw to Units
  In Bus Element : Inport  PortName=RawSensorData  Element=Euler_raw
  In Bus Element1 : Inport  PortName=RawSensorData  Element=Ab_raw
  In Bus Element2 : Inport  PortName=RawSensorData  Element=G_raw
  In Bus Element3 : Inport  PortName=RawSensorData  Element=q_raw
  In Bus Element4 : Inport  PortName=RawSensorData  Element=static_raw
  In Bus Element5 : Inport  PortName=RawSensorData  Element=T_raw
  In Bus Element6 : Inport  PortName=RawSensorData  Element=ctrlSurface_PWM
  1D Discrete Filter : mbdriLib/Filtering/1D Discrete Filter  bw=sensors.antialiasBW  TSample=ap.apSampleTime
      settings: AttributesFormatString=Fc = 40
  1D Discrete Filter1 : mbdriLib/Filtering/1D Discrete Filter  bw=sensors.antialiasBW  TSample=ap.apSampleTime
      settings: AttributesFormatString=Fc = 40
  1D Discrete Filter2 : mbdriLib/Filtering/1D Discrete Filter  bw=sensors.antialiasBW  TSample=ap.apSampleTime
      settings: AttributesFormatString=Fc = 40
  3D Discrete Filter : mbdriLib/Filtering/3D Discrete Filter  bw=sensors.antialiasBW  TSample=ap.apSampleTime
      settings: AttributesFormatString=Fc = 40
  3D Discrete Filter1 : mbdriLib/Filtering/3D Discrete Filter  bw=sensors.antialiasBW  TSample=ap.apSampleTime
      settings: AttributesFormatString=Fc = 40
  3D Discrete Filter2 : mbdriLib/Filtering/3D Discrete Filter  bw=sensors.antialiasBW  TSample=ap.apSampleTime
      settings: AttributesFormatString=Fc = 40
  8192 : Gain  Description=8192/1  Gain=sensors.max_temp/sensors.bit_scale  OutDataTypeStr=single
      settings: AttributesFormatString=%<Gain>
  8192*(2pi)^-1 : Gain  Gain=sensors.max_euler/sensors.bit_scale  OutDataTypeStr=single
      settings: AttributesFormatString=%<Gain>
  8192*.025 : Gain  Gain=sensors.max_gyro/sensors.bit_scale  OutDataTypeStr=single
      settings: AttributesFormatString=%<Gain>
  8192*0.5 : Gain  Gain=sensors.max_ctrlSrfc/sensors.bit_scale  OutDataTypeStr=single
      settings: AttributesFormatString=%<Gain>
  8192*4096^-1 : Gain  Gain=sensors.max_dyn/sensors.bit_scale  OutDataTypeStr=single
      settings: AttributesFormatString=%<Gain>
  Ab_g*8192*0.25 : Gain  Gain=sensors.max_accel/sensors.bit_scale  OutDataTypeStr=single
      settings: AttributesFormatString=%<Gain>
  Constant1 : Constant  Value=env.ISA_P0
      settings: AttributesFormatString=%<Value>
  Data Type Conversion{1..3,5..7} (6 alike) : DataTypeConversion  OutDataTypeStr=single
  Gain1 : Gain  Gain=env.ISA_g  OutDataTypeStr=single
      settings: AttributesFormatString=%<Gain>
  Signal Specification : SignalSpecification  OutDataTypeStr=single  Unit=K
  Signal Specification1 : SignalSpecification  OutDataTypeStr=single  Unit=Pa
  Sum : Sum  Inputs=|-+
  Out Bus Element : Outport  VectorParamsAs1DForOutWhenUnconnected=off  PortName=FilteredSensorData  Element=Euler
  Out Bus Element1 : Outport  VectorParamsAs1DForOutWhenUnconnected=off  PortName=FilteredSensorData  Element=Ab
  Out Bus Element2 : Outport  VectorParamsAs1DForOutWhenUnconnected=off  PortName=FilteredSensorData  Element=G
  Out Bus Element3 : Outport  VectorParamsAs1DForOutWhenUnconnected=off  PortName=FilteredSensorData  Element=q
  Out Bus Element4 : Outport  VectorParamsAs1DForOutWhenUnconnected=off  PortName=FilteredSensorData  Element=baro
  Out Bus Element5 : Outport  VectorParamsAs1DForOutWhenUnconnected=off  PortName=FilteredSensorData  Element=T
  CtrlSurfaces : Outport  Port=2  VectorParamsAs1DForOutWhenUnconnected=off
  wires:
  8192*0.5/1 -> Data Type Conversion3/1  "ctrlSurfaces_rad"
  In Bus Element6/1 -> 8192*0.5/1
  Data Type Conversion3/1 -> CtrlSurfaces/1
  1D Discrete Filter2/1 -> Signal Specification/1
  Data Type Conversion2/1 -> Out Bus Element4/1
  1D Discrete Filter1/1 -> Data Type Conversion2/1
  1D Discrete Filter/1 -> Signal Specification1/1
  3D Discrete Filter2/1 -> Data Type Conversion7/1
  3D Discrete Filter1/1 -> Data Type Conversion5/1
  3D Discrete Filter/1 -> Data Type Conversion6/1
  Data Type Conversion1/1 -> Sum/1
  Gain1/1 -> 3D Discrete Filter1/1
  In Bus Element1/1 -> Ab_g*8192*0.25/1
  Data Type Conversion6/1 -> Out Bus Element/1
  Data Type Conversion5/1 -> Out Bus Element1/1
  Data Type Conversion7/1 -> Out Bus Element2/1
  Signal Specification1/1 -> Out Bus Element3/1
  Sum/1 -> 1D Discrete Filter1/1
  Signal Specification/1 -> Out Bus Element5/1
  Constant1/1 -> Sum/2
  8192/1 -> 1D Discrete Filter2/1
  8192*4096^-1/1 -> 1D Discrete Filter/1
  In Bus Element5/1 -> 8192/1
  In Bus Element4/1 -> Data Type Conversion1/1
  In Bus Element3/1 -> 8192*4096^-1/1
  In Bus Element2/1 -> 8192*.025/1
  8192*.025/1 -> 3D Discrete Filter2/1
  8192*(2pi)^-1/1 -> 3D Discrete Filter/1
  Ab_g*8192*0.25/1 -> Gain1/1
  In Bus Element/1 -> 8192*(2pi)^-1/1

== system FixedWingModel/FixedWingModel/HighFidelity/FixedWingNoWindNoNoise/FixedWingAutopilotModel/Sensor Module/apStatusCreation ==
  In Bus Element7 : Inport  PortName=PosVel_hat  Element=Xe_hat
  In Bus Element8 : Inport  PortName=PosVel_hat  Element=Ve_hat
  In Bus Element10 : Inport  Port=2  PortName=GPSData
  In Bus Element9 : Inport  Port=2  PortName=GPSData  Element=gps_h
  In Bus Element : Inport  Port=3  PortName=FilteredSensorData  Element=Ab
  In Bus Element1 : Inport  Port=3  PortName=FilteredSensorData  Element=G
  In Bus Element2 : Inport  Port=3  PortName=FilteredSensorData  Element=Euler
  In Bus Element3 : Inport  Port=3  PortName=FilteredSensorData  Element=baro
  In Bus Element4 : Inport  Port=3  PortName=FilteredSensorData  Element=q
  Air Density from Height : mbdriLib/Air Utilities/Air Density from Height  SystemSampleTime=-1  VariantActivationTime=update diagram  Latency=0  AutoFrameSizeCalculation=off
  Bus Creator1 : BusCreator  Inputs=8  OutDataTypeStr=Bus: apStatusBus  NonVirtualBus=on
  Compute Airspeed : mbdriLib/Air Utilities/Compute Airspeed  SystemSampleTime=-1  VariantActivationTime=update diagram  Latency=0  AutoFrameSizeCalculation=off
  apStatus : Outport  VectorParamsAs1DForOutWhenUnconnected=off
  wires:
  In Bus Element1/1 -> Bus Creator1/2  "G"
  In Bus Element/1 -> Bus Creator1/1  "Ab"
  In Bus Element10/1 -> Bus Creator1/8  "GPS"
  In Bus Element2/1 -> Bus Creator1/3  "Euler"
  Compute Airspeed/1 -> Bus Creator1/4  "ias"
  Air Density from Height/1 -> Compute Airspeed/2
  In Bus Element8/1 -> Bus Creator1/7  "Ve"
  Bus Creator1/1 -> apStatus/1
  In Bus Element4/1 -> Compute Airspeed/1
  In Bus Element3/1 -> Bus Creator1/5  "baro"
  In Bus Element7/1 -> Bus Creator1/6  "Xe"
  In Bus Element9/1 -> Air Density from Height/1

== system FixedWingModel/FixedWingModel/HighFidelity/FixedWingNoWindNoNoise/FixedWingAutopilotModel/InnerLoopAutopilot/Latch Trim Conditions/Latch Control Surfaces Trim from any mode ==
  ctrlSurfaces : Inport
  Trigger : TriggerPort  TriggerType=falling  VariantControl=Variant
  Trim : Outport  VectorParamsAs1DForOutWhenUnconnected=off
  wires:
  ctrlSurfaces/1 -> Trim/1

== system FixedWingModel/FixedWingModel/HighFidelity/FixedWingNoWindNoNoise/FixedWingAutopilotModel/InnerLoopAutopilot/Longitudinal Channel/Compute Feed Forward ==
  dEFFGain : Inport
  SensorData : Inport  Port=2
  1D Discrete Filter : mbdriLib/Filtering/1D Discrete Filter  bw=10  TSample=ap.apSampleTime
      settings: AttributesFormatString=Fc = 10
  Add5 : Sum  Inputs=+-  OutDataTypeStr=single
  Bus Selector : BusSelector  OutputSignals=Euler
  Constant2 : Constant  OutDataTypeStr=single
      settings: AttributesFormatString=%<Value>
  Constant4 : Constant  OutDataTypeStr=single
      settings: AttributesFormatString=%<Value>
  Product : Product  Inputs=*/  RndMeth=Zero
  Product1 : Product  RndMeth=Zero
  Selector : Selector  InputPortWidth=3  IndexOptions=Index vector (dialog)  Indices=[1]  OutputSizes=1
  Trigonometric Function : Trigonometry  Operator=cos
  "[-60 60]" : Saturate  UpperLimit=60  LowerLimit=-60
      settings: AttributesFormatString="[%<LowerLimit>  %<UpperLimit>]"
  FF : Outport  VectorParamsAs1DForOutWhenUnconnected=off
  wires:
  Selector/1 -> 1D Discrete Filter/1
  Product/1 -> Add5/1
  Constant4/1 -> Product/1
  1D Discrete Filter/1 -> "[-60 60]"/1
  Trigonometric Function/1 -> Product/2
  Constant2/1 -> Add5/2
  Product1/1 -> FF/1
  Add5/1 -> Product1/2
  "[-60 60]"/1 -> Trigonometric Function/1
  Bus Selector/1 -> Selector/1  "<Euler>"
  dEFFGain/1 -> Product1/1
  SensorData/1 -> Bus Selector/1

== system FixedWingModel/FixedWingModel/HighFidelity/FixedWingNoWindNoNoise/FixedWingAutopilotModel/InnerLoopAutopilot/Longitudinal Channel/Height Error to Pitch Command [PI] ==
  Error : Inport
  Reset : Inport  Port=2
  PIDGains : Inport  Port=3
  Demux : Demux  Outputs=3
  PID Controller : pid_lib/PID Controller  Controller=PI  Form=Parallel  TimeDomain=Discrete-time  UseExternalTs=off  SampleTime=ap.apSampleTime  IntegratorMethod=Trapezoidal  FilterMethod=Forward Euler  ControllerParametersSource=external  P=1  I=1  D=0  UseFilter=on  N=100  TunerSelectOption=Transfer Function Based (PID Tuner App)  InitialConditionSource=internal  InitialConditionForIntegrator=0  InitialConditionForFilter=0  DifferentiatorICPrevScaledInput=0  ExternalReset=level  TrackingMode=off  Kt=1  LimitOutput=on  SatLimitsSource=internal  UpperSaturationLimit=ap.control.the_cLimit  LowerSaturationLimit=-ap.control.the_cLimit  LinearizeAsGain=on  AntiWindupMode=clamping  Kb=1  POutMin=[]  POutMax=[]  IOutMin=[]  IOutMax=[]  DOutMin=[]  DOutMax=[]  NOutMin=[]  NOutMax=[]  SumOutMin=[]  SumOutMax=[]  SaturationOutMin=[]  SaturationOutMax=[]  PParamMin=[]  PParamMax=[]  IParamMin=[]  IParamMax=[]  DParamMin=[]  DParamMax=[]  NParamMin=[]  NParamMax=[]  KbParamMin=[]  KbParamMax=[]  KtParamMin=[]  KtParamMax=[]  KbOutMin=[]  KbOutMax=[]  KtOutMin=[]  KtOutMax=[]  IntegratorOutMin=[]  IntegratorOutMax=[]  FilterOutMin=[]  FilterOutMax=[]  SumI1OutMin=[]  SumI1OutMax=[]  SumI2OutMin=[]  SumI2OutMax=[]  SumI3OutMin=[]  SumI3OutMax=[]  SumI4OutMin=[]  SumI4OutMax=[]  SumDOutMin=[]  SumDOutMax=[]  DifferentiatorOutMin=[]  DifferentiatorOutMax=[]  FilterDiffOutCoefMin=[]  FilterDiffOutCoefMax=[]  ReciprocalOutMin=[]  ReciprocalOutMax=[]  SumDenOutMin=[]  SumDenOutMax=[]  SumNumOutMin=[]  SumNumOutMax=[]  DivideOutMin=[]  DivideOutMax=[]  UdiffTsProdOutMin=[]  UdiffTsProdOutMax=[]  NTsProdOutMin=[]  NTsProdOutMax=[]  UintegralTsProdOutMin=[]  UintegralTsProdOutMax=[]  UngainTsProdOutMin=[]  UngainTsProdOutMax=[]  IntegratorContinuousStateAttributes=''  IntegratorStateMustResolveToSignalObject=off  IntegratorRTWStateStorageClass=Auto  FilterContinuousStateAttributes=''  FilterStateMustResolveToSignalObject=off  FilterRTWStateStorageClass=Auto  ParallelPVariant=ExternalParameters  IdealPVariant=Disabled  IVariant=ExternalParameters  DVariant=Disabled  IntegratorVariant=Discrete  SatVariant=Enabled  AWVariant=DiscClampingParallel  PCopyVariant=Disabled  TRVariant=Disabled  FdbkBlocksVariant=Feedback  IdealPFdbkVariant=Passthrough  SatFdbkVariant=Passthrough  DerivativeFilterVariant=Disabled  NVariant=Disabled  NCopyVariant=Disabled_SignalSpec  FilterICVariant=Disabled  IntegratorICVariant=InternalICs  ExternalResetVariant=ExternalReset  TRSumVariant=Passthrough  SumFdbkVariant=Enabled  SumVariant=Sum_PI  TsampFilterVariant=InternalTs  TsampNgainVariant=Passthrough  TsampIntegralVariant=Passthrough  ExternalSaturationOutDataTypeStr=Inherit: Same as second input
  Terminator : Terminator
  Output : Outport  VectorParamsAs1DForOutWhenUnconnected=off
  wires:
  Demux/3 -> Terminator/1
  Error/1 -> PID Controller/1
  PIDGains/1 -> Demux/1
  Demux/1 -> PID Controller/2
  Demux/2 -> PID Controller/3
  Reset/1 -> PID Controller/4
  PID Controller/1 -> Output/1

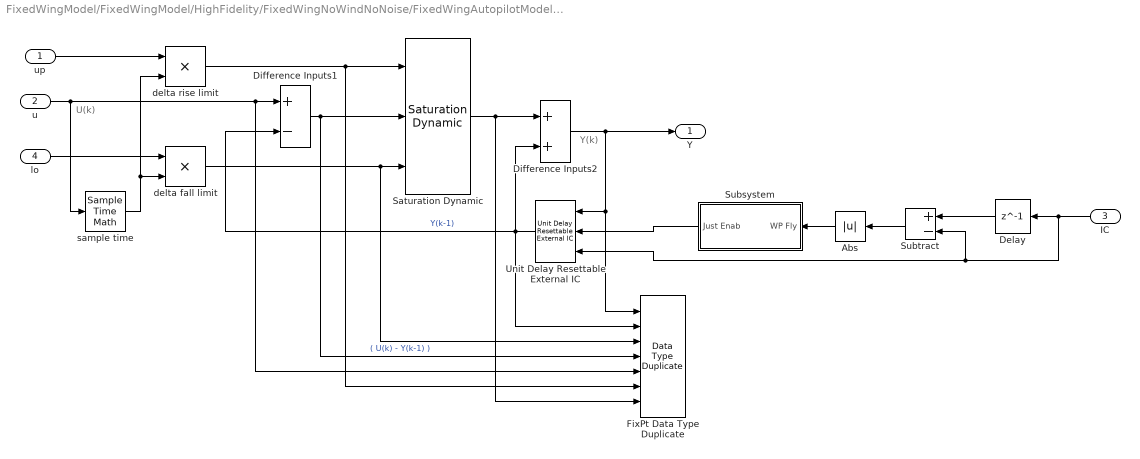
== system FixedWingModel/FixedWingModel/HighFidelity/FixedWingNoWindNoNoise/FixedWingAutopilotModel/InnerLoopAutopilot/Longitudinal Channel/Rate Limiter Dynamic with External IC and Autoreset for Change in IC ==
  note: Y(k)
  note: U(k)
  up : Inport
  u : Inport  Port=2
  IC : Inport  Port=3
  lo : Inport  Port=4
  Abs : Abs
  Delay : Delay  DelayLength=1
  Difference Inputs1 : Sum  Description=Add in CPU  DisableCoverage=on  Inputs=+-  OutDataTypeStr=Inherit: Inherit via back propagation
  Difference Inputs2 : Sum  Description=Add in CPU  OutDataTypeStr=Inherit: Inherit via back propagation
  FixPt Data Type Duplicate : DataTypeDuplicate  DisableCoverage=on  NumInputPorts=7
  Saturation Dynamic : simulink/Discontinuities/Saturation Dynamic  OutMin=[]  OutMax=[]  OutDataTypeStr=Inherit: Same as second input  OutDataType=fixdt(1, 16)  OutScaling=2^-10  DoSatur=off
  Subsystem : Subsystem
  Subtract : Sum  Inputs=+-
  Unit Delay Resettable External IC : simulink_need_slupdate/Unit Delay Resettable External IC  tsamp=-1
      settings: SourceProductBaseCode=SL
  delta fall limit : Product  DisableCoverage=on  Inputs=**  OutDataTypeStr=Inherit: Inherit via back propagation  SaturateOnIntegerOverflow=on
  delta rise limit : Product  DisableCoverage=on  Inputs=**  OutDataTypeStr=Inherit: Inherit via back propagation  SaturateOnIntegerOverflow=on
  sample time : SampleTimeMath  DisableCoverage=on  TsampMathOp=Ts Only  weightValue=1
  Y : Outport  VectorParamsAs1DForOutWhenUnconnected=off
  wires:
  Abs/1 -> Subsystem/1(WP Fly)
  Subsystem/1(Just Enab) -> Unit Delay Resettable External IC/2
  Subtract/1 -> Abs/1
  IC/1 -> Delay/1, Subtract/2, Unit Delay Resettable External IC/3
  Delay/1 -> Subtract/1
  sample time/1 -> delta fall limit/2, delta rise limit/2
  lo/1 -> delta fall limit/1
  delta rise limit/1 -> FixPt Data Type Duplicate/6, Saturation Dynamic/1
  up/1 -> delta rise limit/1
  Difference Inputs2/1 -> FixPt Data Type Duplicate/1, Unit Delay Resettable External IC/1, Y/1
  Unit Delay Resettable External IC/1 -> Difference Inputs1/2, FixPt Data Type Duplicate/2, Difference Inputs2/2  "Y(k-1)"
  Saturation Dynamic/1 -> Difference Inputs2/1, FixPt Data Type Duplicate/7
  delta fall limit/1 -> FixPt Data Type Duplicate/3, Saturation Dynamic/3
  u/1 -> Difference Inputs1/1, FixPt Data Type Duplicate/5, sample time/1
  Difference Inputs1/1 -> FixPt Data Type Duplicate/4, Saturation Dynamic/2  "( U(k) - Y(k-1) )"

== system FixedWingModel/FixedWingModel/HighFidelity/FixedWingNoWindNoNoise/FixedWingAutopilotModel/Sensor Module/Position Filter/Baro Altimeter ==
  Static (Pa) : Inport
  Constant : Constant  Value=101325
      settings: AttributesFormatString=%<Value>
  Constant1 : Constant  Value=-8.31432
      settings: AttributesFormatString=%<Value>
  Constant2 : Constant  Value=288.15
      settings: AttributesFormatString=%<Value>
  Constant3 : Constant  Value=0.0289644
      settings: AttributesFormatString=%<Value>
  Constant4 : Constant  Value=env.ISA_g
      settings: AttributesFormatString=%<Value>
  Divide : Product  Inputs=*/
  Math Function : Math  Operator=log  SignedPower=on  SaturateOnIntegerOverflow=on
  Product : Product  Inputs=***//
  "[80k - 120k]" : Saturate  UpperLimit=160000  LowerLimit=80000
      settings: AttributesFormatString="[%<LowerLimit>  %<UpperLimit>]"
  Altitude : Outport  VectorParamsAs1DForOutWhenUnconnected=off
  wires:
  Product/1 -> Altitude/1
  Constant4/1 -> Product/5
  Constant3/1 -> Product/4
  Constant2/1 -> Product/3
  Constant1/1 -> Product/2
  Math Function/1 -> Product/1
  Divide/1 -> Math Function/1
  "[80k - 120k]"/1 -> Divide/1
  Constant/1 -> Divide/2
  Static (Pa)/1 -> "[80k - 120k]"/1

== system FixedWingModel/FixedWingModel/HighFidelity/FixedWingNoWindNoNoise/FixedWingAutopilotModel/Sensor Module/Position Filter/GPS Update ==
  note: If any of the coordinates have changed, set output to 1
  Xe : Inport
  Detect Change : simulink/Logic and Bit Operations/Detect Change  vinit=0  OutDataTypeStr=boolean
  Logical Operator : Logic  Operator=OR  Inputs=1  AllPortsSameDT=off  OutDataTypeStr=boolean
  Update? : Outport  VectorParamsAs1DForOutWhenUnconnected=off
  wires:
  Xe/1 -> Detect Change/1
  Detect Change/1 -> Logical Operator/1
  Logical Operator/1 -> Update?/1

== system FixedWingModel/FixedWingModel/HighFidelity/FixedWingNoWindNoNoise/FixedWingAutopilotModel/Sensor Module/Position Filter/Get Vn Ve ==
  COG : Inport
  SOG : Inport  Port=2
  Angle Conversion : aerolibconvert2/Angle Conversion  IU=deg  OU=rad
  Product : Product  RndMeth=Zero
  Product1 : Product  RndMeth=Zero
  Subsystem5 : Subsystem
  Vnorth : Outport  Unit=m/s  VectorParamsAs1DForOutWhenUnconnected=off
  Veast : Outport  Port=2  Unit=m/s  VectorParamsAs1DForOutWhenUnconnected=off
  wires:
  Product1/1 -> Vnorth/1
  Product/1 -> Veast/1
  SOG/1 -> Product1/1, Product/2
  Angle Conversion/1 -> Subsystem5/1(u)
  Subsystem5/1(sin(u)) -> Product/1
  Subsystem5/2(cos(u)) -> Product1/2
  COG/1 -> Angle Conversion/1

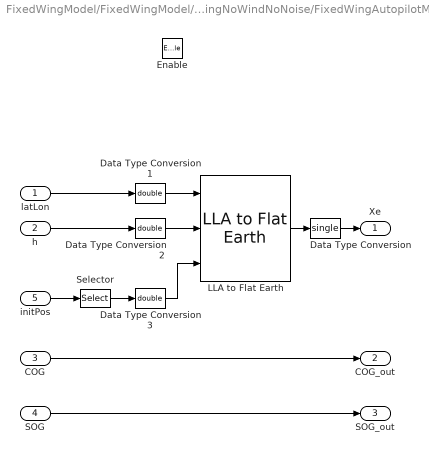
== system FixedWingModel/FixedWingModel/HighFidelity/FixedWingNoWindNoNoise/FixedWingAutopilotModel/Sensor Module/Position Filter/LLA to Flat Earth ==
  latLon : Inport
  h : Inport  Port=2
  COG : Inport  Port=3
  SOG : Inport  Port=4
  initPos : Inport  Port=5
  Enable : EnablePort
  Data Type Conversion : DataTypeConversion  OutDataTypeStr=single
  Data Type Conversion1 : DataTypeConversion  OutDataTypeStr=double
  Data Type Conversion2 : DataTypeConversion  OutDataTypeStr=double
  Data Type Conversion3 : DataTypeConversion  OutDataTypeStr=double
  LLA to Flat Earth : aerolibtransform2/LLA to Flat Earth  units=Metric (MKS)  ptype=Earth (WGS84)  F=1/298.257223563  R=6378137  refPosPort=off  LL0=uavParam.ic.gsLL  psi=0
      settings: SourceProductBaseCode=AE
  Selector : Selector  InputPortWidth=3  IndexOptions=Index vector (dialog)  Indices=[3]  OutputSizes=1
  Xe : Outport  VectorParamsAs1DForOutWhenUnconnected=off
  COG_out : Outport  Port=2  VectorParamsAs1DForOutWhenUnconnected=off
  SOG_out : Outport  Port=3  VectorParamsAs1DForOutWhenUnconnected=off
  wires:
  SOG/1 -> SOG_out/1
  COG/1 -> COG_out/1
  Selector/1 -> Data Type Conversion3/1
  latLon/1 -> Data Type Conversion1/1
  initPos/1 -> Selector/1
  h/1 -> Data Type Conversion2/1
  LLA to Flat Earth/1 -> Data Type Conversion/1
  Data Type Conversion1/1 -> LLA to Flat Earth/1
  Data Type Conversion2/1 -> LLA to Flat Earth/2
  Data Type Conversion3/1 -> LLA to Flat Earth/3
  Data Type Conversion/1 -> Xe/1
